simulink model "ppfir5"  (R2012b)
settings: Solver=VariableStepDiscrete  SolverMode=SingleTasking  StartTime=0.0  StopTime=10000  RelTol=1e-3
libraries: xbsIndex_r4 x8411, casper_library_misc x82, xps_library x6
(part 36 of 79)

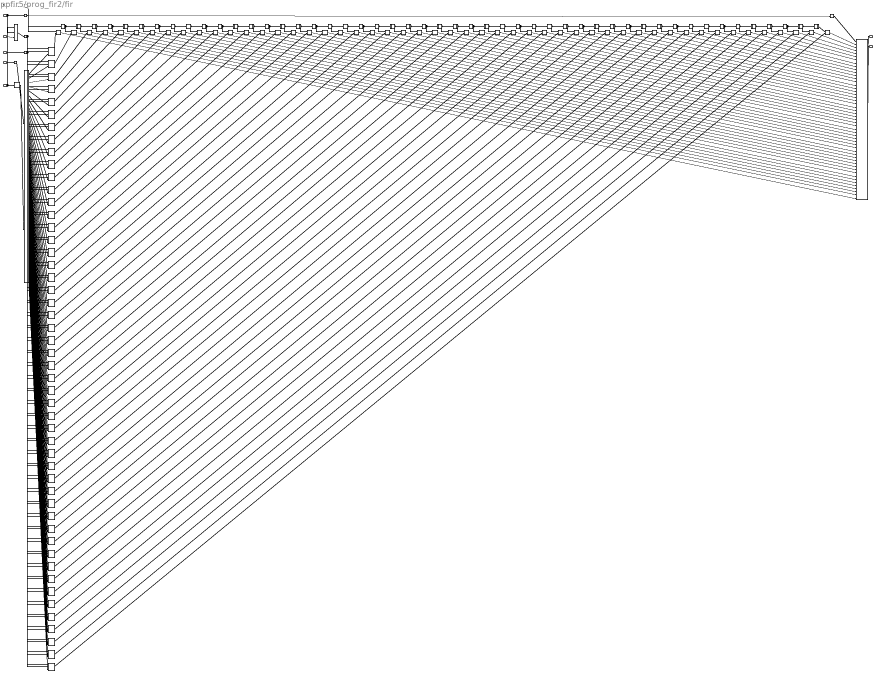
== system ppfir5/prog_fir2/fir ==
  data_in : Inport
  ch_in : Inport  Port=2
  write_coeff : Inport  Port=3
  coeff_to_write : Inport  Port=4
  tap_to_write : Inport  Port=5
  ch_to_write : Inport  Port=6
  Mult{1..50} (50 alike) : xbsIndex_r4/Mult  precision=Full  arith_type="Signed  (2's comp)"  n_bits=16  bin_pt=14  quantization=Truncate  overflow=Wrap  en=off  latency=4  dbl_ovrd=off  use_behavioral_HDL=off  opt=Speed  use_embedded=on  optimum_pipeline=on  pipeline=on  use_rpm=on  placement_style=Triangular  block_type=mult
  bram{1..50} (50 alike) : xbsIndex_r4/Single Port RAM  depth=256  initVector=0  distributed_mem=Block RAM  write_mode=No Read On Write  rst=off  init_reg=0  en=off  latency=3  dbl_ovrd=off  optimize=Area  block_type=spram
  ch_dly : xbsIndex_r4/Delay  rst=off  infoeditControl=Selection of Reset will increase slice count due to use of real FFs and instead of SRLs  en=off  latency=2  dbl_ovrd=off  reg_retiming=off  block_type=delay
  ch_mux : xbsIndex_r4/Mux  inputs=2  en=off  latency=1  precision=Full  arith_type=Unsigned  n_bits=16  bin_pt=14  quantization=Truncate  overflow=Wrap  dbl_ovrd=off  block_type=mux
  coeff_in_dly : xbsIndex_r4/Delay  rst=off  infoeditControl=Selection of Reset will increase slice count due to use of real FFs and instead of SRLs  en=off  latency=3  dbl_ovrd=off  reg_retiming=off  block_type=delay
  data_dly : xbsIndex_r4/Delay  rst=off  infoeditControl=Selection of Reset will increase slice count due to use of real FFs and instead of SRLs  en=off  latency=6  dbl_ovrd=off  reg_retiming=off  block_type=delay
  delay1 : Subsystem  mask(delay_bram){DelayLen=256, bram_latency=2, implementation=Fabric, async=off}
      mask prompts: DelayLen "Delay By:"; bram_latency "BRAM Latency"; implementation "Implement using"; async "asynchronous operation"
      mask help: A delay block that uses BRAM for its storage.
      mask init:
      | delay_bram_impl_init(gcb, ...
      |     'DelayLen', DelayLen, ...
      |     'bram_latency', bram_latency, ...
      |     'implementation', implementation, ...
      |     'async', async);
      mask Help: eval('xlWeb(''http://casper.berkeley.edu/wiki/Delay_bram'')')
      mask TypeOptions implementation: Behavioral HDL | Fabric | DSP48
      mask Display:
      | str=sprintf('z^{-%d}',DelayLen);
      | color('black');disp(str,'texmode','on');
  delay10 : Subsystem  mask(delay_bram){DelayLen=256, bram_latency=2, implementation=Fabric, async=off}
      mask prompts: DelayLen "Delay By:"; bram_latency "BRAM Latency"; implementation "Implement using"; async "asynchronous operation"
      mask help: A delay block that uses BRAM for its storage.
      mask init:
      | delay_bram_impl_init(gcb, ...
      |     'DelayLen', DelayLen, ...
      |     'bram_latency', bram_latency, ...
      |     'implementation', implementation, ...
      |     'async', async);
      mask Help: eval('xlWeb(''http://casper.berkeley.edu/wiki/Delay_bram'')')
      mask TypeOptions implementation: Behavioral HDL | Fabric | DSP48
      mask Display:
      | str=sprintf('z^{-%d}',DelayLen);
      | color('black');disp(str,'texmode','on');
  delay11 : Subsystem  mask(delay_bram){DelayLen=256, bram_latency=2, implementation=Fabric, async=off}
      mask prompts: DelayLen "Delay By:"; bram_latency "BRAM Latency"; implementation "Implement using"; async "asynchronous operation"
      mask help: A delay block that uses BRAM for its storage.
      mask init:
      | delay_bram_impl_init(gcb, ...
      |     'DelayLen', DelayLen, ...
      |     'bram_latency', bram_latency, ...
      |     'implementation', implementation, ...
      |     'async', async);
      mask Help: eval('xlWeb(''http://casper.berkeley.edu/wiki/Delay_bram'')')
      mask TypeOptions implementation: Behavioral HDL | Fabric | DSP48
      mask Display:
      | str=sprintf('z^{-%d}',DelayLen);
      | color('black');disp(str,'texmode','on');
  delay12 : Subsystem  mask(delay_bram){DelayLen=256, bram_latency=2, implementation=Fabric, async=off}
      mask prompts: DelayLen "Delay By:"; bram_latency "BRAM Latency"; implementation "Implement using"; async "asynchronous operation"
      mask help: A delay block that uses BRAM for its storage.
      mask init:
      | delay_bram_impl_init(gcb, ...
      |     'DelayLen', DelayLen, ...
      |     'bram_latency', bram_latency, ...
      |     'implementation', implementation, ...
      |     'async', async);
      mask Help: eval('xlWeb(''http://casper.berkeley.edu/wiki/Delay_bram'')')
      mask TypeOptions implementation: Behavioral HDL | Fabric | DSP48
      mask Display:
      | str=sprintf('z^{-%d}',DelayLen);
      | color('black');disp(str,'texmode','on');
  delay13 : Subsystem  mask(delay_bram){DelayLen=256, bram_latency=2, implementation=Fabric, async=off}
      mask prompts: DelayLen "Delay By:"; bram_latency "BRAM Latency"; implementation "Implement using"; async "asynchronous operation"
      mask help: A delay block that uses BRAM for its storage.
      mask init:
      | delay_bram_impl_init(gcb, ...
      |     'DelayLen', DelayLen, ...
      |     'bram_latency', bram_latency, ...
      |     'implementation', implementation, ...
      |     'async', async);
      mask Help: eval('xlWeb(''http://casper.berkeley.edu/wiki/Delay_bram'')')
      mask TypeOptions implementation: Behavioral HDL | Fabric | DSP48
      mask Display:
      | str=sprintf('z^{-%d}',DelayLen);
      | color('black');disp(str,'texmode','on');
  delay14 : Subsystem  mask(delay_bram){DelayLen=256, bram_latency=2, implementation=Fabric, async=off}
      mask prompts: DelayLen "Delay By:"; bram_latency "BRAM Latency"; implementation "Implement using"; async "asynchronous operation"
      mask help: A delay block that uses BRAM for its storage.
      mask init:
      | delay_bram_impl_init(gcb, ...
      |     'DelayLen', DelayLen, ...
      |     'bram_latency', bram_latency, ...
      |     'implementation', implementation, ...
      |     'async', async);
      mask Help: eval('xlWeb(''http://casper.berkeley.edu/wiki/Delay_bram'')')
      mask TypeOptions implementation: Behavioral HDL | Fabric | DSP48
      mask Display:
      | str=sprintf('z^{-%d}',DelayLen);
      | color('black');disp(str,'texmode','on');
  delay15 : Subsystem  mask(delay_bram){DelayLen=256, bram_latency=2, implementation=Fabric, async=off}
      mask prompts: DelayLen "Delay By:"; bram_latency "BRAM Latency"; implementation "Implement using"; async "asynchronous operation"
      mask help: A delay block that uses BRAM for its storage.
      mask init:
      | delay_bram_impl_init(gcb, ...
      |     'DelayLen', DelayLen, ...
      |     'bram_latency', bram_latency, ...
      |     'implementation', implementation, ...
      |     'async', async);
      mask Help: eval('xlWeb(''http://casper.berkeley.edu/wiki/Delay_bram'')')
      mask TypeOptions implementation: Behavioral HDL | Fabric | DSP48
      mask Display:
      | str=sprintf('z^{-%d}',DelayLen);
      | color('black');disp(str,'texmode','on');
  delay16 : Subsystem  mask(delay_bram){DelayLen=256, bram_latency=2, implementation=Fabric, async=off}
      mask prompts: DelayLen "Delay By:"; bram_latency "BRAM Latency"; implementation "Implement using"; async "asynchronous operation"
      mask help: A delay block that uses BRAM for its storage.
      mask init:
      | delay_bram_impl_init(gcb, ...
      |     'DelayLen', DelayLen, ...
      |     'bram_latency', bram_latency, ...
      |     'implementation', implementation, ...
      |     'async', async);
      mask Help: eval('xlWeb(''http://casper.berkeley.edu/wiki/Delay_bram'')')
      mask TypeOptions implementation: Behavioral HDL | Fabric | DSP48
      mask Display:
      | str=sprintf('z^{-%d}',DelayLen);
      | color('black');disp(str,'texmode','on');
  delay17 : Subsystem  mask(delay_bram){DelayLen=256, bram_latency=2, implementation=Fabric, async=off}
      mask prompts: DelayLen "Delay By:"; bram_latency "BRAM Latency"; implementation "Implement using"; async "asynchronous operation"
      mask help: A delay block that uses BRAM for its storage.
      mask init:
      | delay_bram_impl_init(gcb, ...
      |     'DelayLen', DelayLen, ...
      |     'bram_latency', bram_latency, ...
      |     'implementation', implementation, ...
      |     'async', async);
      mask Help: eval('xlWeb(''http://casper.berkeley.edu/wiki/Delay_bram'')')
      mask TypeOptions implementation: Behavioral HDL | Fabric | DSP48
      mask Display:
      | str=sprintf('z^{-%d}',DelayLen);
      | color('black');disp(str,'texmode','on');
  delay18 : Subsystem  mask(delay_bram){DelayLen=256, bram_latency=2, implementation=Fabric, async=off}
      mask prompts: DelayLen "Delay By:"; bram_latency "BRAM Latency"; implementation "Implement using"; async "asynchronous operation"
      mask help: A delay block that uses BRAM for its storage.
      mask init:
      | delay_bram_impl_init(gcb, ...
      |     'DelayLen', DelayLen, ...
      |     'bram_latency', bram_latency, ...
      |     'implementation', implementation, ...
      |     'async', async);
      mask Help: eval('xlWeb(''http://casper.berkeley.edu/wiki/Delay_bram'')')
      mask TypeOptions implementation: Behavioral HDL | Fabric | DSP48
      mask Display:
      | str=sprintf('z^{-%d}',DelayLen);
      | color('black');disp(str,'texmode','on');
  delay19 : Subsystem  mask(delay_bram){DelayLen=256, bram_latency=2, implementation=Fabric, async=off}
      mask prompts: DelayLen "Delay By:"; bram_latency "BRAM Latency"; implementation "Implement using"; async "asynchronous operation"
      mask help: A delay block that uses BRAM for its storage.
      mask init:
      | delay_bram_impl_init(gcb, ...
      |     'DelayLen', DelayLen, ...
      |     'bram_latency', bram_latency, ...
      |     'implementation', implementation, ...
      |     'async', async);
      mask Help: eval('xlWeb(''http://casper.berkeley.edu/wiki/Delay_bram'')')
      mask TypeOptions implementation: Behavioral HDL | Fabric | DSP48
      mask Display:
      | str=sprintf('z^{-%d}',DelayLen);
      | color('black');disp(str,'texmode','on');
  delay2 : Subsystem  mask(delay_bram){DelayLen=256, bram_latency=2, implementation=Fabric, async=off}
      mask prompts: DelayLen "Delay By:"; bram_latency "BRAM Latency"; implementation "Implement using"; async "asynchronous operation"
      mask help: A delay block that uses BRAM for its storage.
      mask init:
      | delay_bram_impl_init(gcb, ...
      |     'DelayLen', DelayLen, ...
      |     'bram_latency', bram_latency, ...
      |     'implementation', implementation, ...
      |     'async', async);
      mask Help: eval('xlWeb(''http://casper.berkeley.edu/wiki/Delay_bram'')')
      mask TypeOptions implementation: Behavioral HDL | Fabric | DSP48
      mask Display:
      | str=sprintf('z^{-%d}',DelayLen);
      | color('black');disp(str,'texmode','on');
  delay20 : Subsystem  mask(delay_bram){DelayLen=256, bram_latency=2, implementation=Fabric, async=off}
      mask prompts: DelayLen "Delay By:"; bram_latency "BRAM Latency"; implementation "Implement using"; async "asynchronous operation"
      mask help: A delay block that uses BRAM for its storage.
      mask init:
      | delay_bram_impl_init(gcb, ...
      |     'DelayLen', DelayLen, ...
      |     'bram_latency', bram_latency, ...
      |     'implementation', implementation, ...
      |     'async', async);
      mask Help: eval('xlWeb(''http://casper.berkeley.edu/wiki/Delay_bram'')')
      mask TypeOptions implementation: Behavioral HDL | Fabric | DSP48
      mask Display:
      | str=sprintf('z^{-%d}',DelayLen);
      | color('black');disp(str,'texmode','on');
  delay21 : Subsystem  mask(delay_bram){DelayLen=256, bram_latency=2, implementation=Fabric, async=off}
      mask prompts: DelayLen "Delay By:"; bram_latency "BRAM Latency"; implementation "Implement using"; async "asynchronous operation"
      mask help: A delay block that uses BRAM for its storage.
      mask init:
      | delay_bram_impl_init(gcb, ...
      |     'DelayLen', DelayLen, ...
      |     'bram_latency', bram_latency, ...
      |     'implementation', implementation, ...
      |     'async', async);
      mask Help: eval('xlWeb(''http://casper.berkeley.edu/wiki/Delay_bram'')')
      mask TypeOptions implementation: Behavioral HDL | Fabric | DSP48
      mask Display:
      | str=sprintf('z^{-%d}',DelayLen);
      | color('black');disp(str,'texmode','on');
  delay22 : Subsystem  mask(delay_bram){DelayLen=256, bram_latency=2, implementation=Fabric, async=off}
      mask prompts: DelayLen "Delay By:"; bram_latency "BRAM Latency"; implementation "Implement using"; async "asynchronous operation"
      mask help: A delay block that uses BRAM for its storage.
      mask init:
      | delay_bram_impl_init(gcb, ...
      |     'DelayLen', DelayLen, ...
      |     'bram_latency', bram_latency, ...
      |     'implementation', implementation, ...
      |     'async', async);
      mask Help: eval('xlWeb(''http://casper.berkeley.edu/wiki/Delay_bram'')')
      mask TypeOptions implementation: Behavioral HDL | Fabric | DSP48
      mask Display:
      | str=sprintf('z^{-%d}',DelayLen);
      | color('black');disp(str,'texmode','on');
  delay23 : Subsystem  mask(delay_bram){DelayLen=256, bram_latency=2, implementation=Fabric, async=off}
      mask prompts: DelayLen "Delay By:"; bram_latency "BRAM Latency"; implementation "Implement using"; async "asynchronous operation"
      mask help: A delay block that uses BRAM for its storage.
      mask init:
      | delay_bram_impl_init(gcb, ...
      |     'DelayLen', DelayLen, ...
      |     'bram_latency', bram_latency, ...
      |     'implementation', implementation, ...
      |     'async', async);
      mask Help: eval('xlWeb(''http://casper.berkeley.edu/wiki/Delay_bram'')')
      mask TypeOptions implementation: Behavioral HDL | Fabric | DSP48
      mask Display:
      | str=sprintf('z^{-%d}',DelayLen);
      | color('black');disp(str,'texmode','on');
  delay24 : Subsystem  mask(delay_bram){DelayLen=256, bram_latency=2, implementation=Fabric, async=off}
      mask prompts: DelayLen "Delay By:"; bram_latency "BRAM Latency"; implementation "Implement using"; async "asynchronous operation"
      mask help: A delay block that uses BRAM for its storage.
      mask init:
      | delay_bram_impl_init(gcb, ...
      |     'DelayLen', DelayLen, ...
      |     'bram_latency', bram_latency, ...
      |     'implementation', implementation, ...
      |     'async', async);
      mask Help: eval('xlWeb(''http://casper.berkeley.edu/wiki/Delay_bram'')')
      mask TypeOptions implementation: Behavioral HDL | Fabric | DSP48
      mask Display:
      | str=sprintf('z^{-%d}',DelayLen);
      | color('black');disp(str,'texmode','on');
  delay25 : Subsystem  mask(delay_bram){DelayLen=256, bram_latency=2, implementation=Fabric, async=off}
      mask prompts: DelayLen "Delay By:"; bram_latency "BRAM Latency"; implementation "Implement using"; async "asynchronous operation"
      mask help: A delay block that uses BRAM for its storage.
      mask init:
      | delay_bram_impl_init(gcb, ...
      |     'DelayLen', DelayLen, ...
      |     'bram_latency', bram_latency, ...
      |     'implementation', implementation, ...
      |     'async', async);
      mask Help: eval('xlWeb(''http://casper.berkeley.edu/wiki/Delay_bram'')')
      mask TypeOptions implementation: Behavioral HDL | Fabric | DSP48
      mask Display:
      | str=sprintf('z^{-%d}',DelayLen);
      | color('black');disp(str,'texmode','on');
  delay26 : Subsystem  mask(delay_bram){DelayLen=256, bram_latency=2, implementation=Fabric, async=off}
      mask prompts: DelayLen "Delay By:"; bram_latency "BRAM Latency"; implementation "Implement using"; async "asynchronous operation"
      mask help: A delay block that uses BRAM for its storage.
      mask init:
      | delay_bram_impl_init(gcb, ...
      |     'DelayLen', DelayLen, ...
      |     'bram_latency', bram_latency, ...
      |     'implementation', implementation, ...
      |     'async', async);
      mask Help: eval('xlWeb(''http://casper.berkeley.edu/wiki/Delay_bram'')')
      mask TypeOptions implementation: Behavioral HDL | Fabric | DSP48
      mask Display:
      | str=sprintf('z^{-%d}',DelayLen);
      | color('black');disp(str,'texmode','on');
  delay27 : Subsystem  mask(delay_bram){DelayLen=256, bram_latency=2, implementation=Fabric, async=off}
      mask prompts: DelayLen "Delay By:"; bram_latency "BRAM Latency"; implementation "Implement using"; async "asynchronous operation"
      mask help: A delay block that uses BRAM for its storage.
      mask init:
      | delay_bram_impl_init(gcb, ...
      |     'DelayLen', DelayLen, ...
      |     'bram_latency', bram_latency, ...
      |     'implementation', implementation, ...
      |     'async', async);
      mask Help: eval('xlWeb(''http://casper.berkeley.edu/wiki/Delay_bram'')')
      mask TypeOptions implementation: Behavioral HDL | Fabric | DSP48
      mask Display:
      | str=sprintf('z^{-%d}',DelayLen);
      | color('black');disp(str,'texmode','on');
  delay28 : Subsystem  mask(delay_bram){DelayLen=256, bram_latency=2, implementation=Fabric, async=off}
      mask prompts: DelayLen "Delay By:"; bram_latency "BRAM Latency"; implementation "Implement using"; async "asynchronous operation"
      mask help: A delay block that uses BRAM for its storage.
      mask init:
      | delay_bram_impl_init(gcb, ...
      |     'DelayLen', DelayLen, ...
      |     'bram_latency', bram_latency, ...
      |     'implementation', implementation, ...
      |     'async', async);
      mask Help: eval('xlWeb(''http://casper.berkeley.edu/wiki/Delay_bram'')')
      mask TypeOptions implementation: Behavioral HDL | Fabric | DSP48
      mask Display:
      | str=sprintf('z^{-%d}',DelayLen);
      | color('black');disp(str,'texmode','on');
  delay29 : Subsystem  mask(delay_bram){DelayLen=256, bram_latency=2, implementation=Fabric, async=off}
      mask prompts: DelayLen "Delay By:"; bram_latency "BRAM Latency"; implementation "Implement using"; async "asynchronous operation"
      mask help: A delay block that uses BRAM for its storage.
      mask init:
      | delay_bram_impl_init(gcb, ...
      |     'DelayLen', DelayLen, ...
      |     'bram_latency', bram_latency, ...
      |     'implementation', implementation, ...
      |     'async', async);
      mask Help: eval('xlWeb(''http://casper.berkeley.edu/wiki/Delay_bram'')')
      mask TypeOptions implementation: Behavioral HDL | Fabric | DSP48
      mask Display:
      | str=sprintf('z^{-%d}',DelayLen);
      | color('black');disp(str,'texmode','on');
  delay3 : Subsystem  mask(delay_bram){DelayLen=256, bram_latency=2, implementation=Fabric, async=off}
      mask prompts: DelayLen "Delay By:"; bram_latency "BRAM Latency"; implementation "Implement using"; async "asynchronous operation"
      mask help: A delay block that uses BRAM for its storage.
      mask init:
      | delay_bram_impl_init(gcb, ...
      |     'DelayLen', DelayLen, ...
      |     'bram_latency', bram_latency, ...
      |     'implementation', implementation, ...
      |     'async', async);
      mask Help: eval('xlWeb(''http://casper.berkeley.edu/wiki/Delay_bram'')')
      mask TypeOptions implementation: Behavioral HDL | Fabric | DSP48
      mask Display:
      | str=sprintf('z^{-%d}',DelayLen);
      | color('black');disp(str,'texmode','on');
  delay30 : Subsystem  mask(delay_bram){DelayLen=256, bram_latency=2, implementation=Fabric, async=off}
      mask prompts: DelayLen "Delay By:"; bram_latency "BRAM Latency"; implementation "Implement using"; async "asynchronous operation"
      mask help: A delay block that uses BRAM for its storage.
      mask init:
      | delay_bram_impl_init(gcb, ...
      |     'DelayLen', DelayLen, ...
      |     'bram_latency', bram_latency, ...
      |     'implementation', implementation, ...
      |     'async', async);
      mask Help: eval('xlWeb(''http://casper.berkeley.edu/wiki/Delay_bram'')')
      mask TypeOptions implementation: Behavioral HDL | Fabric | DSP48
      mask Display:
      | str=sprintf('z^{-%d}',DelayLen);
      | color('black');disp(str,'texmode','on');
  delay31 : Subsystem  mask(delay_bram){DelayLen=256, bram_latency=2, implementation=Fabric, async=off}
      mask prompts: DelayLen "Delay By:"; bram_latency "BRAM Latency"; implementation "Implement using"; async "asynchronous operation"
      mask help: A delay block that uses BRAM for its storage.
      mask init:
      | delay_bram_impl_init(gcb, ...
      |     'DelayLen', DelayLen, ...
      |     'bram_latency', bram_latency, ...
      |     'implementation', implementation, ...
      |     'async', async);
      mask Help: eval('xlWeb(''http://casper.berkeley.edu/wiki/Delay_bram'')')
      mask TypeOptions implementation: Behavioral HDL | Fabric | DSP48
      mask Display:
      | str=sprintf('z^{-%d}',DelayLen);
      | color('black');disp(str,'texmode','on');
  delay32 : Subsystem  mask(delay_bram){DelayLen=256, bram_latency=2, implementation=Fabric, async=off}
      mask prompts: DelayLen "Delay By:"; bram_latency "BRAM Latency"; implementation "Implement using"; async "asynchronous operation"
      mask help: A delay block that uses BRAM for its storage.
      mask init:
      | delay_bram_impl_init(gcb, ...
      |     'DelayLen', DelayLen, ...
      |     'bram_latency', bram_latency, ...
      |     'implementation', implementation, ...
      |     'async', async);
      mask Help: eval('xlWeb(''http://casper.berkeley.edu/wiki/Delay_bram'')')
      mask TypeOptions implementation: Behavioral HDL | Fabric | DSP48
      mask Display:
      | str=sprintf('z^{-%d}',DelayLen);
      | color('black');disp(str,'texmode','on');
  delay33 : Subsystem  mask(delay_bram){DelayLen=256, bram_latency=2, implementation=Fabric, async=off}
      mask prompts: DelayLen "Delay By:"; bram_latency "BRAM Latency"; implementation "Implement using"; async "asynchronous operation"
      mask help: A delay block that uses BRAM for its storage.
      mask init:
      | delay_bram_impl_init(gcb, ...
      |     'DelayLen', DelayLen, ...
      |     'bram_latency', bram_latency, ...
      |     'implementation', implementation, ...
      |     'async', async);
      mask Help: eval('xlWeb(''http://casper.berkeley.edu/wiki/Delay_bram'')')
      mask TypeOptions implementation: Behavioral HDL | Fabric | DSP48
      mask Display:
      | str=sprintf('z^{-%d}',DelayLen);
      | color('black');disp(str,'texmode','on');
  delay34 : Subsystem  mask(delay_bram){DelayLen=256, bram_latency=2, implementation=Fabric, async=off}
      mask prompts: DelayLen "Delay By:"; bram_latency "BRAM Latency"; implementation "Implement using"; async "asynchronous operation"
      mask help: A delay block that uses BRAM for its storage.
      mask init:
      | delay_bram_impl_init(gcb, ...
      |     'DelayLen', DelayLen, ...
      |     'bram_latency', bram_latency, ...
      |     'implementation', implementation, ...
      |     'async', async);
      mask Help: eval('xlWeb(''http://casper.berkeley.edu/wiki/Delay_bram'')')
      mask TypeOptions implementation: Behavioral HDL | Fabric | DSP48
      mask Display:
      | str=sprintf('z^{-%d}',DelayLen);
      | color('black');disp(str,'texmode','on');
  delay35 : Subsystem  mask(delay_bram){DelayLen=256, bram_latency=2, implementation=Fabric, async=off}
      mask prompts: DelayLen "Delay By:"; bram_latency "BRAM Latency"; implementation "Implement using"; async "asynchronous operation"
      mask help: A delay block that uses BRAM for its storage.
      mask init:
      | delay_bram_impl_init(gcb, ...
      |     'DelayLen', DelayLen, ...
      |     'bram_latency', bram_latency, ...
      |     'implementation', implementation, ...
      |     'async', async);
      mask Help: eval('xlWeb(''http://casper.berkeley.edu/wiki/Delay_bram'')')
      mask TypeOptions implementation: Behavioral HDL | Fabric | DSP48
      mask Display:
      | str=sprintf('z^{-%d}',DelayLen);
      | color('black');disp(str,'texmode','on');
  delay36 : Subsystem  mask(delay_bram){DelayLen=256, bram_latency=2, implementation=Fabric, async=off}
      mask prompts: DelayLen "Delay By:"; bram_latency "BRAM Latency"; implementation "Implement using"; async "asynchronous operation"
      mask help: A delay block that uses BRAM for its storage.
      mask init:
      | delay_bram_impl_init(gcb, ...
      |     'DelayLen', DelayLen, ...
      |     'bram_latency', bram_latency, ...
      |     'implementation', implementation, ...
      |     'async', async);
      mask Help: eval('xlWeb(''http://casper.berkeley.edu/wiki/Delay_bram'')')
      mask TypeOptions implementation: Behavioral HDL | Fabric | DSP48
      mask Display:
      | str=sprintf('z^{-%d}',DelayLen);
      | color('black');disp(str,'texmode','on');
  delay37 : Subsystem  mask(delay_bram){DelayLen=256, bram_latency=2, implementation=Fabric, async=off}
      mask prompts: DelayLen "Delay By:"; bram_latency "BRAM Latency"; implementation "Implement using"; async "asynchronous operation"
      mask help: A delay block that uses BRAM for its storage.
      mask init:
      | delay_bram_impl_init(gcb, ...
      |     'DelayLen', DelayLen, ...
      |     'bram_latency', bram_latency, ...
      |     'implementation', implementation, ...
      |     'async', async);
      mask Help: eval('xlWeb(''http://casper.berkeley.edu/wiki/Delay_bram'')')
      mask TypeOptions implementation: Behavioral HDL | Fabric | DSP48
      mask Display:
      | str=sprintf('z^{-%d}',DelayLen);
      | color('black');disp(str,'texmode','on');
  delay38 : Subsystem  mask(delay_bram){DelayLen=256, bram_latency=2, implementation=Fabric, async=off}
      mask prompts: DelayLen "Delay By:"; bram_latency "BRAM Latency"; implementation "Implement using"; async "asynchronous operation"
      mask help: A delay block that uses BRAM for its storage.
      mask init:
      | delay_bram_impl_init(gcb, ...
      |     'DelayLen', DelayLen, ...
      |     'bram_latency', bram_latency, ...
      |     'implementation', implementation, ...
      |     'async', async);
      mask Help: eval('xlWeb(''http://casper.berkeley.edu/wiki/Delay_bram'')')
      mask TypeOptions implementation: Behavioral HDL | Fabric | DSP48
      mask Display:
      | str=sprintf('z^{-%d}',DelayLen);
      | color('black');disp(str,'texmode','on');
  delay39 : Subsystem  mask(delay_bram){DelayLen=256, bram_latency=2, implementation=Fabric, async=off}
      mask prompts: DelayLen "Delay By:"; bram_latency "BRAM Latency"; implementation "Implement using"; async "asynchronous operation"
      mask help: A delay block that uses BRAM for its storage.
      mask init:
      | delay_bram_impl_init(gcb, ...
      |     'DelayLen', DelayLen, ...
      |     'bram_latency', bram_latency, ...
      |     'implementation', implementation, ...
      |     'async', async);
      mask Help: eval('xlWeb(''http://casper.berkeley.edu/wiki/Delay_bram'')')
      mask TypeOptions implementation: Behavioral HDL | Fabric | DSP48
      mask Display:
      | str=sprintf('z^{-%d}',DelayLen);
      | color('black');disp(str,'texmode','on');
  delay4 : Subsystem  mask(delay_bram){DelayLen=256, bram_latency=2, implementation=Fabric, async=off}
      mask prompts: DelayLen "Delay By:"; bram_latency "BRAM Latency"; implementation "Implement using"; async "asynchronous operation"
      mask help: A delay block that uses BRAM for its storage.
      mask init:
      | delay_bram_impl_init(gcb, ...
      |     'DelayLen', DelayLen, ...
      |     'bram_latency', bram_latency, ...
      |     'implementation', implementation, ...
      |     'async', async);
      mask Help: eval('xlWeb(''http://casper.berkeley.edu/wiki/Delay_bram'')')
      mask TypeOptions implementation: Behavioral HDL | Fabric | DSP48
      mask Display:
      | str=sprintf('z^{-%d}',DelayLen);
      | color('black');disp(str,'texmode','on');
  delay40 : Subsystem  mask(delay_bram){DelayLen=256, bram_latency=2, implementation=Fabric, async=off}
      mask prompts: DelayLen "Delay By:"; bram_latency "BRAM Latency"; implementation "Implement using"; async "asynchronous operation"
      mask help: A delay block that uses BRAM for its storage.
      mask init:
      | delay_bram_impl_init(gcb, ...
      |     'DelayLen', DelayLen, ...
      |     'bram_latency', bram_latency, ...
      |     'implementation', implementation, ...
      |     'async', async);
      mask Help: eval('xlWeb(''http://casper.berkeley.edu/wiki/Delay_bram'')')
      mask TypeOptions implementation: Behavioral HDL | Fabric | DSP48
      mask Display:
      | str=sprintf('z^{-%d}',DelayLen);
      | color('black');disp(str,'texmode','on');
  delay41 : Subsystem  mask(delay_bram){DelayLen=256, bram_latency=2, implementation=Fabric, async=off}
      mask prompts: DelayLen "Delay By:"; bram_latency "BRAM Latency"; implementation "Implement using"; async "asynchronous operation"
      mask help: A delay block that uses BRAM for its storage.
      mask init:
      | delay_bram_impl_init(gcb, ...
      |     'DelayLen', DelayLen, ...
      |     'bram_latency', bram_latency, ...
      |     'implementation', implementation, ...
      |     'async', async);
      mask Help: eval('xlWeb(''http://casper.berkeley.edu/wiki/Delay_bram'')')
      mask TypeOptions implementation: Behavioral HDL | Fabric | DSP48
      mask Display:
      | str=sprintf('z^{-%d}',DelayLen);
      | color('black');disp(str,'texmode','on');
  delay42 : Subsystem  mask(delay_bram){DelayLen=256, bram_latency=2, implementation=Fabric, async=off}
      mask prompts: DelayLen "Delay By:"; bram_latency "BRAM Latency"; implementation "Implement using"; async "asynchronous operation"
      mask help: A delay block that uses BRAM for its storage.
      mask init:
      | delay_bram_impl_init(gcb, ...
      |     'DelayLen', DelayLen, ...
      |     'bram_latency', bram_latency, ...
      |     'implementation', implementation, ...
      |     'async', async);
      mask Help: eval('xlWeb(''http://casper.berkeley.edu/wiki/Delay_bram'')')
      mask TypeOptions implementation: Behavioral HDL | Fabric | DSP48
      mask Display:
      | str=sprintf('z^{-%d}',DelayLen);
      | color('black');disp(str,'texmode','on');
  delay43 : Subsystem  mask(delay_bram){DelayLen=256, bram_latency=2, implementation=Fabric, async=off}
      mask prompts: DelayLen "Delay By:"; bram_latency "BRAM Latency"; implementation "Implement using"; async "asynchronous operation"
      mask help: A delay block that uses BRAM for its storage.
      mask init:
      | delay_bram_impl_init(gcb, ...
      |     'DelayLen', DelayLen, ...
      |     'bram_latency', bram_latency, ...
      |     'implementation', implementation, ...
      |     'async', async);
      mask Help: eval('xlWeb(''http://casper.berkeley.edu/wiki/Delay_bram'')')
      mask TypeOptions implementation: Behavioral HDL | Fabric | DSP48
      mask Display:
      | str=sprintf('z^{-%d}',DelayLen);
      | color('black');disp(str,'texmode','on');
  delay44 : Subsystem  mask(delay_bram){DelayLen=256, bram_latency=2, implementation=Fabric, async=off}
      mask prompts: DelayLen "Delay By:"; bram_latency "BRAM Latency"; implementation "Implement using"; async "asynchronous operation"
      mask help: A delay block that uses BRAM for its storage.
      mask init:
      | delay_bram_impl_init(gcb, ...
      |     'DelayLen', DelayLen, ...
      |     'bram_latency', bram_latency, ...
      |     'implementation', implementation, ...
      |     'async', async);
      mask Help: eval('xlWeb(''http://casper.berkeley.edu/wiki/Delay_bram'')')
      mask TypeOptions implementation: Behavioral HDL | Fabric | DSP48
      mask Display:
      | str=sprintf('z^{-%d}',DelayLen);
      | color('black');disp(str,'texmode','on');
  delay45 : Subsystem  mask(delay_bram){DelayLen=256, bram_latency=2, implementation=Fabric, async=off}
      mask prompts: DelayLen "Delay By:"; bram_latency "BRAM Latency"; implementation "Implement using"; async "asynchronous operation"
      mask help: A delay block that uses BRAM for its storage.
      mask init:
      | delay_bram_impl_init(gcb, ...
      |     'DelayLen', DelayLen, ...
      |     'bram_latency', bram_latency, ...
      |     'implementation', implementation, ...
      |     'async', async);
      mask Help: eval('xlWeb(''http://casper.berkeley.edu/wiki/Delay_bram'')')
      mask TypeOptions implementation: Behavioral HDL | Fabric | DSP48
      mask Display:
      | str=sprintf('z^{-%d}',DelayLen);
      | color('black');disp(str,'texmode','on');
  delay46 : Subsystem  mask(delay_bram){DelayLen=256, bram_latency=2, implementation=Fabric, async=off}
      mask prompts: DelayLen "Delay By:"; bram_latency "BRAM Latency"; implementation "Implement using"; async "asynchronous operation"
      mask help: A delay block that uses BRAM for its storage.
      mask init:
      | delay_bram_impl_init(gcb, ...
      |     'DelayLen', DelayLen, ...
      |     'bram_latency', bram_latency, ...
      |     'implementation', implementation, ...
      |     'async', async);
      mask Help: eval('xlWeb(''http://casper.berkeley.edu/wiki/Delay_bram'')')
      mask TypeOptions implementation: Behavioral HDL | Fabric | DSP48
      mask Display:
      | str=sprintf('z^{-%d}',DelayLen);
      | color('black');disp(str,'texmode','on');
  delay47 : Subsystem  mask(delay_bram){DelayLen=256, bram_latency=2, implementation=Fabric, async=off}
      mask prompts: DelayLen "Delay By:"; bram_latency "BRAM Latency"; implementation "Implement using"; async "asynchronous operation"
      mask help: A delay block that uses BRAM for its storage.
      mask init:
      | delay_bram_impl_init(gcb, ...
      |     'DelayLen', DelayLen, ...
      |     'bram_latency', bram_latency, ...
      |     'implementation', implementation, ...
      |     'async', async);
      mask Help: eval('xlWeb(''http://casper.berkeley.edu/wiki/Delay_bram'')')
      mask TypeOptions implementation: Behavioral HDL | Fabric | DSP48
      mask Display:
      | str=sprintf('z^{-%d}',DelayLen);
      | color('black');disp(str,'texmode','on');
  delay48 : Subsystem  mask(delay_bram){DelayLen=256, bram_latency=2, implementation=Fabric, async=off}
      mask prompts: DelayLen "Delay By:"; bram_latency "BRAM Latency"; implementation "Implement using"; async "asynchronous operation"
      mask help: A delay block that uses BRAM for its storage.
      mask init:
      | delay_bram_impl_init(gcb, ...
      |     'DelayLen', DelayLen, ...
      |     'bram_latency', bram_latency, ...
      |     'implementation', implementation, ...
      |     'async', async);
      mask Help: eval('xlWeb(''http://casper.berkeley.edu/wiki/Delay_bram'')')
      mask TypeOptions implementation: Behavioral HDL | Fabric | DSP48
      mask Display:
      | str=sprintf('z^{-%d}',DelayLen);
      | color('black');disp(str,'texmode','on');
  delay49 : Subsystem  mask(delay_bram){DelayLen=256, bram_latency=2, implementation=Fabric, async=off}
      mask prompts: DelayLen "Delay By:"; bram_latency "BRAM Latency"; implementation "Implement using"; async "asynchronous operation"
      mask help: A delay block that uses BRAM for its storage.
      mask init:
      | delay_bram_impl_init(gcb, ...
      |     'DelayLen', DelayLen, ...
      |     'bram_latency', bram_latency, ...
      |     'implementation', implementation, ...
      |     'async', async);
      mask Help: eval('xlWeb(''http://casper.berkeley.edu/wiki/Delay_bram'')')
      mask TypeOptions implementation: Behavioral HDL | Fabric | DSP48
      mask Display:
      | str=sprintf('z^{-%d}',DelayLen);
      | color('black');disp(str,'texmode','on');
  delay5 : Subsystem  mask(delay_bram){DelayLen=256, bram_latency=2, implementation=Fabric, async=off}
      mask prompts: DelayLen "Delay By:"; bram_latency "BRAM Latency"; implementation "Implement using"; async "asynchronous operation"
      mask help: A delay block that uses BRAM for its storage.
      mask init:
      | delay_bram_impl_init(gcb, ...
      |     'DelayLen', DelayLen, ...
      |     'bram_latency', bram_latency, ...
      |     'implementation', implementation, ...
      |     'async', async);
      mask Help: eval('xlWeb(''http://casper.berkeley.edu/wiki/Delay_bram'')')
      mask TypeOptions implementation: Behavioral HDL | Fabric | DSP48
      mask Display:
      | str=sprintf('z^{-%d}',DelayLen);
      | color('black');disp(str,'texmode','on');
  delay6 : Subsystem  mask(delay_bram){DelayLen=256, bram_latency=2, implementation=Fabric, async=off}
      mask prompts: DelayLen "Delay By:"; bram_latency "BRAM Latency"; implementation "Implement using"; async "asynchronous operation"
      mask help: A delay block that uses BRAM for its storage.
      mask init:
      | delay_bram_impl_init(gcb, ...
      |     'DelayLen', DelayLen, ...
      |     'bram_latency', bram_latency, ...
      |     'implementation', implementation, ...
      |     'async', async);
      mask Help: eval('xlWeb(''http://casper.berkeley.edu/wiki/Delay_bram'')')
      mask TypeOptions implementation: Behavioral HDL | Fabric | DSP48
      mask Display:
      | str=sprintf('z^{-%d}',DelayLen);
      | color('black');disp(str,'texmode','on');
  delay7 : Subsystem  mask(delay_bram){DelayLen=256, bram_latency=2, implementation=Fabric, async=off}
      mask prompts: DelayLen "Delay By:"; bram_latency "BRAM Latency"; implementation "Implement using"; async "asynchronous operation"
      mask help: A delay block that uses BRAM for its storage.
      mask init:
      | delay_bram_impl_init(gcb, ...
      |     'DelayLen', DelayLen, ...
      |     'bram_latency', bram_latency, ...
      |     'implementation', implementation, ...
      |     'async', async);
      mask Help: eval('xlWeb(''http://casper.berkeley.edu/wiki/Delay_bram'')')
      mask TypeOptions implementation: Behavioral HDL | Fabric | DSP48
      mask Display:
      | str=sprintf('z^{-%d}',DelayLen);
      | color('black');disp(str,'texmode','on');
  delay8 : Subsystem  mask(delay_bram){DelayLen=256, bram_latency=2, implementation=Fabric, async=off}
      mask prompts: DelayLen "Delay By:"; bram_latency "BRAM Latency"; implementation "Implement using"; async "asynchronous operation"
      mask help: A delay block that uses BRAM for its storage.
      mask init:
      | delay_bram_impl_init(gcb, ...
      |     'DelayLen', DelayLen, ...
      |     'bram_latency', bram_latency, ...
      |     'implementation', implementation, ...
      |     'async', async);
      mask Help: eval('xlWeb(''http://casper.berkeley.edu/wiki/Delay_bram'')')
      mask TypeOptions implementation: Behavioral HDL | Fabric | DSP48
      mask Display:
      | str=sprintf('z^{-%d}',DelayLen);
      | color('black');disp(str,'texmode','on');
  delay9 : Subsystem  mask(delay_bram){DelayLen=256, bram_latency=2, implementation=Fabric, async=off}
      mask prompts: DelayLen "Delay By:"; bram_latency "BRAM Latency"; implementation "Implement using"; async "asynchronous operation"
      mask help: A delay block that uses BRAM for its storage.
      mask init:
      | delay_bram_impl_init(gcb, ...
      |     'DelayLen', DelayLen, ...
      |     'bram_latency', bram_latency, ...
      |     'implementation', implementation, ...
      |     'async', async);
      mask Help: eval('xlWeb(''http://casper.berkeley.edu/wiki/Delay_bram'')')
      mask TypeOptions implementation: Behavioral HDL | Fabric | DSP48
      mask Display:
      | str=sprintf('z^{-%d}',DelayLen);
      | color('black');disp(str,'texmode','on');
  demux : Subsystem  mask(demux){nOutputs=50, provideEnable=on}
      mask prompts: nOutputs "number of outputs"; provideEnable "provide enable port"
      mask init:
      | demux_init(gcb,'nOutputs',nOutputs,'provideEnable',provideEnable);
  misc_dly : xbsIndex_r4/Delay  rst=off  infoeditControl=Selection of Reset will increase slice count due to use of real FFs and instead of SRLs  en=off  latency=6  dbl_ovrd=off  reg_retiming=off  block_type=delay
  not_clear : xbsIndex_r4/Inverter  en=off  latency=1  dbl_ovrd=off  block_type=inv
  sum : Subsystem  AncestorBlock=casper_library_misc/adder_tree  mask(adder_tree){n_inputs=50, latency=3, adder_imp=DSP48, first_stage_hdl=on}
      mask prompts: n_inputs "Number of Inputs"; latency "Add Latency"; adder_imp "Adder implementation"; first_stage_hdl "Use behavioural HDL for first stage of adders"
      mask help:
      | Sums all inputs using a tree of adds and delays.
      |
      | Number of inputs: The number of inputs to the block to be summed
      | Add latency: The number of clock cycles to perform one addition (affects timing)..
      | Adder implementation: choice of fabric or DSP48E core, or behavioral HDL
      | Use behavioural HDL for first stage of adders: Causes the first stage of adders to be absorbed into DSP blocks if multipliers precede them (Virtex 5). Overrides Adder implementation
      mask init:
      | adder_tree_init(gcb, ...
      |     'n_inputs', n_inputs, ...
      |     'latency', latency, ...
      |     'adder_imp', adder_imp, ...
      |     'first_stage_hdl', first_stage_hdl);
      settings: AttributesFormatString=latency 18
      mask Help: eval('xlWeb(''http://casper.berkeley.edu/wiki/Adder_tree'')')
      mask TypeOptions adder_imp: Behavioral | Fabric | DSP48
  sync_delay : xbsIndex_r4/Delay  rst=off  infoeditControl=Selection of Reset will increase slice count due to use of real FFs and instead of SRLs  en=off  latency=4  dbl_ovrd=off  reg_retiming=off  block_type=delay
  tap_dly : xbsIndex_r4/Delay  rst=off  infoeditControl=Selection of Reset will increase slice count due to use of real FFs and instead of SRLs  en=off  latency=1  dbl_ovrd=off  reg_retiming=off  block_type=delay
  data_out : Outport
  ch_out : Outport  Port=2
  wires:
  data_dly/1 -> Mult1/1, delay1/1(din)
  data_in/1 -> data_dly/1
  demux/50(out49) -> bram50/3
  bram50/1 -> Mult50/2
  Mult50/1 -> sum/2(din1)
  delay49/1(dout) -> Mult50/1
  demux/49(out48) -> bram49/3
  bram49/1 -> Mult49/2
  Mult49/1 -> sum/3(din2)
  delay48/1(dout) -> delay49/1(din), Mult49/1
  demux/48(out47) -> bram48/3
  bram48/1 -> Mult48/2
  Mult48/1 -> sum/4(din3)
  delay47/1(dout) -> delay48/1(din), Mult48/1
  demux/47(out46) -> bram47/3
  bram47/1 -> Mult47/2
  Mult47/1 -> sum/5(din4)
  delay46/1(dout) -> delay47/1(din), Mult47/1
  demux/46(out45) -> bram46/3
  bram46/1 -> Mult46/2
  Mult46/1 -> sum/6(din5)
  delay45/1(dout) -> delay46/1(din), Mult46/1
  demux/45(out44) -> bram45/3
  bram45/1 -> Mult45/2
  Mult45/1 -> sum/7(din6)
  delay44/1(dout) -> delay45/1(din), Mult45/1
  demux/44(out43) -> bram44/3
  bram44/1 -> Mult44/2
  Mult44/1 -> sum/8(din7)
  delay43/1(dout) -> delay44/1(din), Mult44/1
  demux/43(out42) -> bram43/3
  bram43/1 -> Mult43/2
  Mult43/1 -> sum/9(din8)
  delay42/1(dout) -> delay43/1(din), Mult43/1
  demux/42(out41) -> bram42/3
  bram42/1 -> Mult42/2
  Mult42/1 -> sum/10(din9)
  delay41/1(dout) -> delay42/1(din), Mult42/1
  demux/41(out40) -> bram41/3
  bram41/1 -> Mult41/2
  Mult41/1 -> sum/11(din10)
  delay40/1(dout) -> delay41/1(din), Mult41/1
  demux/40(out39) -> bram40/3
  bram40/1 -> Mult40/2
  Mult40/1 -> sum/12(din11)
  delay39/1(dout) -> delay40/1(din), Mult40/1
  demux/39(out38) -> bram39/3
  bram39/1 -> Mult39/2
  Mult39/1 -> sum/13(din12)
  delay38/1(dout) -> delay39/1(din), Mult39/1
  demux/38(out37) -> bram38/3
  bram38/1 -> Mult38/2
  Mult38/1 -> sum/14(din13)
  delay37/1(dout) -> delay38/1(din), Mult38/1
  demux/37(out36) -> bram37/3
  bram37/1 -> Mult37/2
  Mult37/1 -> sum/15(din14)
  delay36/1(dout) -> delay37/1(din), Mult37/1
  demux/36(out35) -> bram36/3
  bram36/1 -> Mult36/2
  Mult36/1 -> sum/16(din15)
  delay35/1(dout) -> delay36/1(din), Mult36/1
  demux/35(out34) -> bram35/3
  bram35/1 -> Mult35/2
  Mult35/1 -> sum/17(din16)
  delay34/1(dout) -> delay35/1(din), Mult35/1
  demux/34(out33) -> bram34/3
  bram34/1 -> Mult34/2
  Mult34/1 -> sum/18(din17)
  delay33/1(dout) -> delay34/1(din), Mult34/1
  demux/33(out32) -> bram33/3
  bram33/1 -> Mult33/2
  Mult33/1 -> sum/19(din18)
  delay32/1(dout) -> delay33/1(din), Mult33/1
  demux/32(out31) -> bram32/3
  bram32/1 -> Mult32/2
  Mult32/1 -> sum/20(din19)
  delay31/1(dout) -> delay32/1(din), Mult32/1
  demux/31(out30) -> bram31/3
  bram31/1 -> Mult31/2
  Mult31/1 -> sum/21(din20)
  delay30/1(dout) -> delay31/1(din), Mult31/1
  demux/30(out29) -> bram30/3
  bram30/1 -> Mult30/2
  Mult30/1 -> sum/22(din21)
  delay29/1(dout) -> delay30/1(din), Mult30/1
  demux/29(out28) -> bram29/3
  bram29/1 -> Mult29/2
  Mult29/1 -> sum/23(din22)
  delay28/1(dout) -> delay29/1(din), Mult29/1
  demux/28(out27) -> bram28/3
  bram28/1 -> Mult28/2
  Mult28/1 -> sum/24(din23)
  delay27/1(dout) -> delay28/1(din), Mult28/1
  demux/27(out26) -> bram27/3
  bram27/1 -> Mult27/2
  Mult27/1 -> sum/25(din24)
  delay26/1(dout) -> delay27/1(din), Mult27/1
  demux/26(out25) -> bram26/3
  bram26/1 -> Mult26/2
  Mult26/1 -> sum/26(din25)
  delay25/1(dout) -> delay26/1(din), Mult26/1
  demux/25(out24) -> bram25/3
  bram25/1 -> Mult25/2
  Mult25/1 -> sum/27(din26)
  delay24/1(dout) -> delay25/1(din), Mult25/1
  demux/24(out23) -> bram24/3
  bram24/1 -> Mult24/2
  Mult24/1 -> sum/28(din27)
  delay23/1(dout) -> delay24/1(din), Mult24/1
  demux/23(out22) -> bram23/3
  bram23/1 -> Mult23/2
  Mult23/1 -> sum/29(din28)
  delay22/1(dout) -> delay23/1(din), Mult23/1
  demux/22(out21) -> bram22/3
  bram22/1 -> Mult22/2
  Mult22/1 -> sum/30(din29)
  delay21/1(dout) -> delay22/1(din), Mult22/1
  demux/21(out20) -> bram21/3
  bram21/1 -> Mult21/2
  Mult21/1 -> sum/31(din30)
  delay20/1(dout) -> delay21/1(din), Mult21/1
  demux/20(out19) -> bram20/3
  bram20/1 -> Mult20/2
  Mult20/1 -> sum/32(din31)
  delay19/1(dout) -> delay20/1(din), Mult20/1
  demux/19(out18) -> bram19/3
  bram19/1 -> Mult19/2
  Mult19/1 -> sum/33(din32)
  delay18/1(dout) -> delay19/1(din), Mult19/1
  demux/18(out17) -> bram18/3
  bram18/1 -> Mult18/2
  Mult18/1 -> sum/34(din33)
  delay17/1(dout) -> delay18/1(din), Mult18/1
  demux/17(out16) -> bram17/3
  bram17/1 -> Mult17/2
  Mult17/1 -> sum/35(din34)
  delay16/1(dout) -> delay17/1(din), Mult17/1
  demux/16(out15) -> bram16/3
  bram16/1 -> Mult16/2
  Mult16/1 -> sum/36(din35)
  delay15/1(dout) -> delay16/1(din), Mult16/1
  demux/15(out14) -> bram15/3
  bram15/1 -> Mult15/2
  Mult15/1 -> sum/37(din36)
  delay14/1(dout) -> delay15/1(din), Mult15/1
  demux/14(out13) -> bram14/3
  bram14/1 -> Mult14/2
  Mult14/1 -> sum/38(din37)
  delay13/1(dout) -> delay14/1(din), Mult14/1
  demux/13(out12) -> bram13/3
  bram13/1 -> Mult13/2
  Mult13/1 -> sum/39(din38)
  delay12/1(dout) -> delay13/1(din), Mult13/1
  demux/12(out11) -> bram12/3
  bram12/1 -> Mult12/2
  Mult12/1 -> sum/40(din39)
  delay11/1(dout) -> delay12/1(din), Mult12/1
  demux/11(out10) -> bram11/3
  bram11/1 -> Mult11/2
  Mult11/1 -> sum/41(din40)
  delay10/1(dout) -> delay11/1(din), Mult11/1
  demux/10(out9) -> bram10/3
  bram10/1 -> Mult10/2
  Mult10/1 -> sum/42(din41)
  delay9/1(dout) -> delay10/1(din), Mult10/1
  demux/9(out8) -> bram9/3
  bram9/1 -> Mult9/2
  Mult9/1 -> sum/43(din42)
  delay8/1(dout) -> delay9/1(din), Mult9/1
  demux/8(out7) -> bram8/3
  bram8/1 -> Mult8/2
  Mult8/1 -> sum/44(din43)
  delay7/1(dout) -> delay8/1(din), Mult8/1
  demux/7(out6) -> bram7/3
  bram7/1 -> Mult7/2
  Mult7/1 -> sum/45(din44)
  delay6/1(dout) -> delay7/1(din), Mult7/1
  demux/6(out5) -> bram6/3
  bram6/1 -> Mult6/2
  Mult6/1 -> sum/46(din45)
  delay5/1(dout) -> delay6/1(din), Mult6/1
  demux/5(out4) -> bram5/3
  bram5/1 -> Mult5/2
  Mult5/1 -> sum/47(din46)
  delay4/1(dout) -> delay5/1(din), Mult5/1
  demux/4(out3) -> bram4/3
  bram4/1 -> Mult4/2
  Mult4/1 -> sum/48(din47)
  delay3/1(dout) -> delay4/1(din), Mult4/1
  demux/3(out2) -> bram3/3
  bram3/1 -> Mult3/2
  Mult3/1 -> sum/49(din48)
  delay2/1(dout) -> delay3/1(din), Mult3/1
  demux/2(out1) -> bram2/3
  bram2/1 -> Mult2/2
  Mult2/1 -> sum/50(din49)
  delay1/1(dout) -> delay2/1(din), Mult2/1
  demux/1(out0) -> bram1/3
  coeff_in_dly/1 -> bram50/2, bram49/2, bram48/2, bram47/2, bram46/2, bram45/2, bram44/2, bram43/2, bram42/2, bram41/2, bram40/2, bram39/2, bram38/2, bram37/2, bram36/2, bram35/2, bram34/2, bram33/2, bram32/2, bram31/2, bram30/2, bram29/2, bram28/2, bram27/2, bram26/2, bram25/2, bram24/2, bram23/2, bram22/2, bram21/2, bram20/2, bram19/2, bram18/2, bram17/2, bram16/2, bram15/2, bram14/2, bram13/2, bram12/2, bram11/2, bram10/2, bram9/2, bram8/2, bram7/2, bram6/2, bram5/2, bram4/2, bram3/2, bram2/2, bram1/2
  ch_dly/1 -> bram50/1, bram49/1, bram48/1, bram47/1, bram46/1, bram45/1, bram44/1, bram43/1, bram42/1, bram41/1, bram40/1, bram39/1, bram38/1, bram37/1, bram36/1, bram35/1, bram34/1, bram33/1, bram32/1, bram31/1, bram30/1, bram29/1, bram28/1, bram27/1, bram26/1, bram25/1, bram24/1, bram23/1, bram22/1, bram21/1, bram20/1, bram19/1, bram18/1, bram17/1, bram16/1, bram15/1, bram14/1, bram13/1, bram12/1, bram11/1, bram10/1, bram9/1, bram8/1, bram7/1, bram6/1, bram5/1, bram4/1, bram3/1, bram2/1, bram1/1
  bram1/1 -> Mult1/2
  Mult1/1 -> sum/51(din50)
  not_clear/1 -> demux/2(clear)
  tap_dly/1 -> demux/1(in)
  sum/1(sync_out) -> ch_out/1
  sync_delay/1 -> sum/1(sync)
  sum/2(dout) -> data_out/1
  misc_dly/1 -> sync_delay/1
  coeff_to_write/1 -> coeff_in_dly/1
  tap_to_write/1 -> tap_dly/1
  ch_mux/1 -> ch_dly/1
  write_coeff/1 -> not_clear/1, ch_mux/1
  ch_to_write/1 -> ch_mux/3
  ch_in/1 -> ch_mux/2, misc_dly/1
